simulink model "ADMIRE"  (R2021b)
settings: Solver=ode4  StartTime=0.0  StopTime=100  FixedStep=1e-2  RelTol=1e-3
undefined symbols (not defined in the file or in its folder): admireDB, Earth, WGS84
libraries: simulink_extras x112, simulink x27, aerolibutil x4, dspsigops x4, aerolibfltsims x3, sharedtransform x2, aerolibtransform2 x2, aerolibatmos2 x1, matrix_library x1, sharedutil x1, aerolibanimutils x1, vrlib x1
(part 15 of 15)

== system ADMIRE/Aircraft/Aerodynamics/YawMomentCoefficient/MachRegion3/Cymdr/Cymdr_ ==
  angleOfAttack_deg : Inport
  mach_nd : Inport  Port=2
  dR : Inport  Port=3
  qacorr : Inport  Port=4
  CYMDRAM_ALFA_M : Lookup_n-D  BreakpointsForDimension1=admireDB.aerodata_asym_ext.CYMDRAM.breakpoints.M  BreakpointsForDimension2=admireDB.aerodata_asym_ext.CYMDRAM.breakpoints.ALFA  BreakpointsForDimension3=[5, 7]  Table=admireDB.aerodata_asym_ext.CYMDRAM.newTable  ExtrapMethod=Clip  InternalRulePriority=Speed  RndMeth=Simplest  InputSameDT=on
      settings: InputPortMap=u0,u1
  CYMEDR_QA_M : Lookup_n-D  BreakpointsForDimension1=admireDB.aerodata_asym_ext.CYMEDR.breakpoints.M  BreakpointsForDimension2=admireDB.aerodata_asym_ext.CYMEDR.breakpoints.QA  BreakpointsForDimension3=[5, 7]  Table=admireDB.aerodata_asym_ext.CYMEDR.newTable  ExtrapMethod=Clip  InternalRulePriority=Speed  RndMeth=Simplest  InputSameDT=on
      settings: InputPortMap=u0,u1
  Degrees to Radians : simulink_extras/Transformations/Degrees to Radians
  Product : Product  Inputs=***
  Cymdr : Outport
  wires:
  Product/1 -> Cymdr/1
  CYMEDR_QA_M/1 -> Product/3
  qacorr/1 -> CYMEDR_QA_M/2
  mach_nd/1 -> CYMEDR_QA_M/1, CYMDRAM_ALFA_M/1
  Degrees to Radians/1 -> Product/2
  angleOfAttack_deg/1 -> CYMDRAM_ALFA_M/2
  CYMDRAM_ALFA_M/1 -> Product/1
  dR/1 -> Degrees to Radians/1

== system ADMIRE/Aircraft/Aerodynamics/YawMomentCoefficient/MachRegion3/Cymp/Cymp_ ==
  angleOfAttack_deg : Inport
  mach_nd : Inport  Port=2
  qacorr : Inport  Port=3
  pc : Inport  Port=4
  CYMEP_QA_M : Lookup_n-D  BreakpointsForDimension1=admireDB.aerodata_asym_ext.CYMEP.breakpoints.M  BreakpointsForDimension2=admireDB.aerodata_asym_ext.CYMEP.breakpoints.QA  BreakpointsForDimension3=[5, 7]  Table=admireDB.aerodata_asym_ext.CYMEP.newTable  ExtrapMethod=Clip  InternalRulePriority=Speed  RndMeth=Simplest  InputSameDT=on
      settings: InputPortMap=u0,u1
  CYMPAM_ALFA_M : Lookup_n-D  BreakpointsForDimension1=admireDB.aerodata_asym_ext.CYMPAM.breakpoints.M  BreakpointsForDimension2=admireDB.aerodata_asym_ext.CYMPAM.breakpoints.ALFA  BreakpointsForDimension3=[5, 7]  Table=admireDB.aerodata_asym_ext.CYMPAM.newTable  ExtrapMethod=Clip  InternalRulePriority=Speed  RndMeth=Simplest  InputSameDT=on
      settings: InputPortMap=u0,u1
  Product : Product
  Sum : Sum  Inputs=|++
  Cymp : Outport
  wires:
  qacorr/1 -> CYMEP_QA_M/2
  CYMEP_QA_M/1 -> Sum/2
  Sum/1 -> Product/1
  mach_nd/1 -> CYMPAM_ALFA_M/1, CYMEP_QA_M/1
  pc/1 -> Product/2
  Product/1 -> Cymp/1
  angleOfAttack_deg/1 -> CYMPAM_ALFA_M/2
  CYMPAM_ALFA_M/1 -> Sum/1

== system ADMIRE/Aircraft/Aerodynamics/YawMomentCoefficient/MachRegion3/Cymr/Cymr_ ==
  mach_nd : Inport
  angleOfAttack_deg : Inport  Port=2
  dN : Inport  Port=3
  qacorr : Inport  Port=4
  rc : Inport  Port=5
  CYMER_M_QA : Lookup_n-D  BreakpointsForDimension1=admireDB.aerodata_asym_ext.CYMER.breakpoints.QA  BreakpointsForDimension2=admireDB.aerodata_asym_ext.CYMER.breakpoints.M  BreakpointsForDimension3=[5, 7]  Table=admireDB.aerodata_asym_ext.CYMER.newTable  ExtrapMethod=Clip  InternalRulePriority=Speed  RndMeth=Simplest  InputSameDT=on
      settings: InputPortMap=u0,u1
  CYMRAM_M_ALFA_DN : Lookup_n-D  NumberOfTableDimensions=3  BreakpointsForDimension1=admireDB.aerodata_asym_ext.CYMRAM.breakpoints.M  BreakpointsForDimension2=admireDB.aerodata_asym_ext.CYMRAM.breakpoints.ALFA  BreakpointsForDimension3=admireDB.aerodata_asym_ext.CYMRAM.breakpoints.DN  Table=admireDB.aerodata_asym_ext.CYMRAM.newTable  ExtrapMethod=Clip  InternalRulePriority=Speed  RndMeth=Simplest  InputSameDT=on
      settings: InputPortMap=u0,u1,u2
  Product : Product  Inputs=***
  Cymr : Outport
  wires:
  CYMER_M_QA/1 -> Product/3
  qacorr/1 -> CYMER_M_QA/1
  dN/1 -> CYMRAM_M_ALFA_DN/3
  rc/1 -> Product/2
  Product/1 -> Cymr/1
  mach_nd/1 -> CYMRAM_M_ALFA_DN/1, CYMER_M_QA/2
  angleOfAttack_deg/1 -> CYMRAM_M_ALFA_DN/2
  CYMRAM_M_ALFA_DN/1 -> Product/1

== system ADMIRE/Aircraft/Aerodynamics/YawMomentCoefficient/MachRegion4/Cymbcai/Cymbcai_ ==
  CAI : Inport
  angleOfAttack_deg : Inport  Port=2
  angleOfSideslip_deg : Inport  Port=3
  CYMBCAI_CAI_ALFA : Lookup_n-D  BreakpointsForDimension1=admireDB.aerodata_asym_ext.CYMBCAI.breakpoints.ALFA  BreakpointsForDimension2=admireDB.aerodata_asym_ext.CYMBCAI.breakpoints.CAI  BreakpointsForDimension3=[5, 7]  Table=admireDB.aerodata_asym_ext.CYMBCAI.newTable  ExtrapMethod=Clip  InternalRulePriority=Speed  RndMeth=Simplest  InputSameDT=on
      settings: InputPortMap=u0,u1
  Degrees to Radians : simulink_extras/Transformations/Degrees to Radians
  Product : Product  Inputs=**
  Cymbcai : Outport
  wires:
  CAI/1 -> CYMBCAI_CAI_ALFA/2
  angleOfSideslip_deg/1 -> Degrees to Radians/1
  CYMBCAI_CAI_ALFA/1 -> Product/1
  angleOfAttack_deg/1 -> CYMBCAI_CAI_ALFA/1
  Degrees to Radians/1 -> Product/2
  Product/1 -> Cymbcai/1

== system ADMIRE/Aircraft/Aerodynamics/YawMomentCoefficient/MachRegion4/Cymbde/Cymbde_ ==
  angleOfAttack_deg : Inport
  dEI : Inport  Port=2
  angleOfSideslip_deg : Inport  Port=3
  dEY : Inport  Port=4
  eieff : Inport  Port=5
  eoeff : Inport  Port=6
  mach_nd : Inport  Port=7
  Abs : Abs
  CYMBKM_M : Lookup_n-D  NumberOfTableDimensions=1  BreakpointsForDimension1=admireDB.aerodata_asym_ext.CYMBKM.breakpoints.M  BreakpointsForDimension3=[5, 7]  Table=admireDB.aerodata_asym_ext.CYMBKM.newTable  ExtrapMethod=Clip  InternalRulePriority=Speed  RndMeth=Simplest  InputSameDT=on
  CYMDEB_ALFA_DE_BETA : Lookup_n-D  NumberOfTableDimensions=3  BreakpointsForDimension1=admireDB.aerodata_asym_ext.CYMDEB.breakpoints.ALFA  BreakpointsForDimension2=admireDB.aerodata_asym_ext.CYMDEB.breakpoints.DE  BreakpointsForDimension3=admireDB.aerodata_asym_ext.CYMDEB.breakpoints.BETA  Table=admireDB.aerodata_asym_ext.CYMDEB.newTable  ExtrapMethod=Clip  InternalRulePriority=Speed  RndMeth=Simplest  InputSameDT=on
      settings: InputPortMap=u0,u1,u2
  CYMDEB_ALFA_DE_BETA1 : Lookup_n-D  NumberOfTableDimensions=3  BreakpointsForDimension1=admireDB.aerodata_asym_ext.CYMDEB.breakpoints.ALFA  BreakpointsForDimension2=admireDB.aerodata_asym_ext.CYMDEB.breakpoints.DE  BreakpointsForDimension3=admireDB.aerodata_asym_ext.CYMDEB.breakpoints.BETA  Table=admireDB.aerodata_asym_ext.CYMDEB.newTable  ExtrapMethod=Clip  InternalRulePriority=Speed  RndMeth=Simplest  InputSameDT=on
      settings: InputPortMap=u0,u1,u2
  Product : Product  Inputs=**
  Product1 : Product  Inputs=**
  Product2 : Product  Inputs=***
  Sign : Signum
  Sum : Sum  Inputs=|++
  Cymbde : Outport
  wires:
  Product2/1 -> Cymbde/1
  dEI/1 -> CYMDEB_ALFA_DE_BETA/2
  angleOfSideslip_deg/1 -> Abs/1, Sign/1
  CYMDEB_ALFA_DE_BETA/1 -> Product/1
  eieff/1 -> Product/2
  dEY/1 -> CYMDEB_ALFA_DE_BETA1/2
  Abs/1 -> CYMDEB_ALFA_DE_BETA/3, CYMDEB_ALFA_DE_BETA1/3
  angleOfAttack_deg/1 -> CYMDEB_ALFA_DE_BETA/1, CYMDEB_ALFA_DE_BETA1/1
  CYMDEB_ALFA_DE_BETA1/1 -> Product1/1
  eoeff/1 -> Product1/2
  Product/1 -> Sum/1
  Product1/1 -> Sum/2
  Sum/1 -> Product2/1
  Sign/1 -> Product2/2
  CYMBKM_M/1 -> Product2/3
  mach_nd/1 -> CYMBKM_M/1

== system ADMIRE/Aircraft/Aerodynamics/YawMomentCoefficient/MachRegion4/Cymbdle/Cymbdle_ ==
  angleOfAttack_deg : Inport
  dEI : Inport  Port=2
  mach_nd : Inport  Port=3
  dEY : Inport  Port=4
  eieff : Inport  Port=5
  eoeff : Inport  Port=6
  angleOfSideslip_deg : Inport  Port=7
  dLE : Inport  Port=8
  CYMBDLE_ALFA_DE_M : Lookup_n-D  NumberOfTableDimensions=3  BreakpointsForDimension1=admireDB.aerodata_asym_ext.CYMBDLE.breakpoints.ALFA  BreakpointsForDimension2=admireDB.aerodata_asym_ext.CYMBDLE.breakpoints.DE  BreakpointsForDimension3=admireDB.aerodata_asym_ext.CYMBDLE.breakpoints.M  Table=admireDB.aerodata_asym_ext.CYMBDLE.newTable  ExtrapMethod=Clip  InternalRulePriority=Speed  RndMeth=Simplest  InputSameDT=on
      settings: InputPortMap=u0,u1,u2
  CYMBDLE_ALFA_DE_M1 : Lookup_n-D  NumberOfTableDimensions=3  BreakpointsForDimension1=admireDB.aerodata_asym_ext.CYMBDLE.breakpoints.ALFA  BreakpointsForDimension2=admireDB.aerodata_asym_ext.CYMBDLE.breakpoints.DE  BreakpointsForDimension3=admireDB.aerodata_asym_ext.CYMBDLE.breakpoints.M  Table=admireDB.aerodata_asym_ext.CYMBDLE.newTable  ExtrapMethod=Clip  InternalRulePriority=Speed  RndMeth=Simplest  InputSameDT=on
      settings: InputPortMap=u0,u1,u2
  Constant : Constant  Value=1/27
  Degrees to Radians : simulink_extras/Transformations/Degrees to Radians
  Product : Product  Inputs=**
  Product1 : Product  Inputs=**
  Product2 : Product  Inputs=****
  Sum : Sum  Inputs=|++
  Cymbdle : Outport
  wires:
  Product2/1 -> Cymbdle/1
  CYMBDLE_ALFA_DE_M/1 -> Product/1
  dEI/1 -> CYMBDLE_ALFA_DE_M/2
  eieff/1 -> Product/2
  mach_nd/1 -> CYMBDLE_ALFA_DE_M1/3, CYMBDLE_ALFA_DE_M/3
  angleOfAttack_deg/1 -> CYMBDLE_ALFA_DE_M1/1, CYMBDLE_ALFA_DE_M/1
  CYMBDLE_ALFA_DE_M1/1 -> Product1/1
  dEY/1 -> CYMBDLE_ALFA_DE_M1/2
  eoeff/1 -> Product1/2
  Product/1 -> Sum/1
  Product1/1 -> Sum/2
  Sum/1 -> Product2/2
  angleOfSideslip_deg/1 -> Degrees to Radians/1
  Degrees to Radians/1 -> Product2/1
  dLE/1 -> Product2/3
  Constant/1 -> Product2/4

== system ADMIRE/Aircraft/Aerodynamics/YawMomentCoefficient/MachRegion4/Cymbdn/Cymbdn_ ==
  angleOfAttack_deg : Inport
  dN : Inport  Port=2
  angleOfSideslip_deg : Inport  Port=3
  Abs : Abs
  CYMDNB_ALFA_DN_BETA : Lookup_n-D  NumberOfTableDimensions=3  BreakpointsForDimension1=admireDB.aerodata_asym_ext.CYMDNB.breakpoints.ALFA  BreakpointsForDimension2=admireDB.aerodata_asym_ext.CYMDNB.breakpoints.DN  BreakpointsForDimension3=admireDB.aerodata_asym_ext.CYMDNB.breakpoints.BETA  Table=admireDB.aerodata_asym_ext.CYMDNB.newTable  ExtrapMethod=Clip  InternalRulePriority=Speed  RndMeth=Simplest  InputSameDT=on
      settings: InputPortMap=u0,u1,u2
  Product : Product  Inputs=**
  Sign : Signum
  Cymbdn : Outport
  wires:
  Product/1 -> Cymbdn/1
  angleOfSideslip_deg/1 -> Sign/1, Abs/1
  angleOfAttack_deg/1 -> CYMDNB_ALFA_DN_BETA/1
  Sign/1 -> Product/2
  CYMDNB_ALFA_DN_BETA/1 -> Product/1
  dN/1 -> CYMDNB_ALFA_DN_BETA/2
  Abs/1 -> CYMDNB_ALFA_DN_BETA/3

== system ADMIRE/Aircraft/Aerodynamics/YawMomentCoefficient/MachRegion4/Cymbeta/Cymbeta_ ==
  angleOfSideslip_deg : Inport
  angleOfAttack_deg : Inport  Port=2
  mach_nd : Inport  Port=3
  qacorr : Inport  Port=4
  Abs : Abs
  CYMEB_QA_M : Lookup_n-D  BreakpointsForDimension1=admireDB.aerodata_asym_ext.CYMEB.breakpoints.M  BreakpointsForDimension2=admireDB.aerodata_asym_ext.CYMEB.breakpoints.QA  BreakpointsForDimension3=[5, 7]  Table=admireDB.aerodata_asym_ext.CYMEB.newTable  ExtrapMethod=Clip  InternalRulePriority=Speed  RndMeth=Simplest  InputSameDT=on
      settings: InputPortMap=u0,u1
  CYMMAB_BETA_ALFA_M : Lookup_n-D  NumberOfTableDimensions=3  BreakpointsForDimension1=admireDB.aerodata_asym_ext.CYMMAB.breakpoints.BETA  BreakpointsForDimension2=admireDB.aerodata_asym_ext.CYMMAB.breakpoints.ALFA  BreakpointsForDimension3=admireDB.aerodata_asym_ext.CYMMAB.breakpoints.M  Table=admireDB.aerodata_asym_ext.CYMMAB.newTable  ExtrapMethod=Clip  InternalRulePriority=Speed  RndMeth=Simplest  InputSameDT=on
      settings: InputPortMap=u0,u1,u2
  Degrees to Radians : simulink_extras/Transformations/Degrees to Radians
  Product : Product  Inputs=**
  Product1 : Product  Inputs=**
  Sign : Signum
  Sum : Sum  Inputs=|++
  Cymbeta : Outport
  wires:
  CYMMAB_BETA_ALFA_M/1 -> Product/2
  angleOfAttack_deg/1 -> CYMMAB_BETA_ALFA_M/2
  Sign/1 -> Product/1
  Product/1 -> Sum/1
  Sum/1 -> Cymbeta/1
  angleOfSideslip_deg/1 -> Sign/1, Degrees to Radians/1, Abs/1
  mach_nd/1 -> CYMMAB_BETA_ALFA_M/3, CYMEB_QA_M/1
  CYMEB_QA_M/1 -> Product1/1
  qacorr/1 -> CYMEB_QA_M/2
  Degrees to Radians/1 -> Product1/2
  Abs/1 -> CYMMAB_BETA_ALFA_M/1
  Product1/1 -> Sum/2

== system ADMIRE/Aircraft/Aerodynamics/YawMomentCoefficient/MachRegion4/Cymbetad/Cymbetad_ ==
  angleOfAttack_deg : Inport
  mach_nd : Inport  Port=2
  betad : Inport  Port=3
  CYMBDH_ALFA_M : Lookup_n-D  BreakpointsForDimension1=admireDB.aerodata_asym_ext.CYMBDH.breakpoints.M  BreakpointsForDimension2=admireDB.aerodata_asym_ext.CYMBDH.breakpoints.ALFA  BreakpointsForDimension3=[5, 7]  Table=admireDB.aerodata_asym_ext.CYMBDH.newTable  ExtrapMethod=Clip  InternalRulePriority=Speed  RndMeth=Simplest  InputSameDT=on
      settings: InputPortMap=u0,u1
  Product : Product  Inputs=**
  Cymbetad : Outport
  wires:
  mach_nd/1 -> CYMBDH_ALFA_M/1
  angleOfAttack_deg/1 -> CYMBDH_ALFA_M/2
  CYMBDH_ALFA_M/1 -> Product/1
  Product/1 -> Cymbetad/1
  betad/1 -> Product/2

== system ADMIRE/Aircraft/Aerodynamics/YawMomentCoefficient/MachRegion4/Cymblg/Cymblg_ ==
  angleOfSideslip_deg : Inport
  dLG : Inport  Port=2
  angleOfAttack_deg : Inport  Port=3
  CYMBLST_NG_DOOR_ALFA : Lookup_n-D  BreakpointsForDimension1=admireDB.aerodata_asym_ext.CYMBLST.breakpoints.ALFA  BreakpointsForDimension2=admireDB.aerodata_asym_ext.CYMBLST.breakpoints.NG_DOOR  BreakpointsForDimension3=[5, 7]  Table=admireDB.aerodata_asym_ext.CYMBLST.newTable  ExtrapMethod=Clip  InternalRulePriority=Speed  RndMeth=Simplest  InputSameDT=on
      settings: InputPortMap=u0,u1
  Degrees to Radians : simulink_extras/Transformations/Degrees to Radians
  Product : Product  Inputs=3
  Cymblg : Outport
  wires:
  CYMBLST_NG_DOOR_ALFA/1 -> Product/3
  Product/1 -> Cymblg/1
  dLG/1 -> CYMBLST_NG_DOOR_ALFA/2, Product/2
  angleOfSideslip_deg/1 -> Degrees to Radians/1
  angleOfAttack_deg/1 -> CYMBLST_NG_DOOR_ALFA/1
  Degrees to Radians/1 -> Product/1

== system ADMIRE/Aircraft/Aerodynamics/YawMomentCoefficient/MachRegion4/Cymdai/Cymdai_ ==
  dAI : Inport
  angleOfAttack_deg : Inport  Port=2
  dEI : Inport  Port=3
  mach_nd : Inport  Port=4
  eieff : Inport  Port=5
  qacorr : Inport  Port=6
  CYMDA_ALFA_DE_M : Lookup_n-D  NumberOfTableDimensions=3  BreakpointsForDimension1=admireDB.aerodata_asym_ext.CYMDA.breakpoints.ALFA  BreakpointsForDimension2=admireDB.aerodata_asym_ext.CYMDA.breakpoints.DE  BreakpointsForDimension3=admireDB.aerodata_asym_ext.CYMDA.breakpoints.M  Table=admireDB.aerodata_asym_ext.CYMDA.newTable  ExtrapMethod=Clip  InternalRulePriority=Speed  RndMeth=Simplest  InputSameDT=on
      settings: InputPortMap=u0,u1,u2
  CYMEDAI_QA_M : Lookup_n-D  BreakpointsForDimension1=admireDB.aerodata_asym_ext.CYMEDAI.breakpoints.M  BreakpointsForDimension2=admireDB.aerodata_asym_ext.CYMEDAI.breakpoints.QA  BreakpointsForDimension3=[5, 7]  Table=admireDB.aerodata_asym_ext.CYMEDAI.newTable  ExtrapMethod=Clip  InternalRulePriority=Speed  RndMeth=Simplest  InputSameDT=on
      settings: InputPortMap=u0,u1
  Degrees to Radians : simulink_extras/Transformations/Degrees to Radians
  Product1 : Product  Inputs=3
  Product2 : Product  Inputs=**
  Cymdai : Outport
  wires:
  qacorr/1 -> CYMEDAI_QA_M/2
  eieff/1 -> Product1/2
  Product2/1 -> Cymdai/1
  dAI/1 -> Degrees to Radians/1
  dEI/1 -> CYMDA_ALFA_DE_M/2
  mach_nd/1 -> CYMDA_ALFA_DE_M/3, CYMEDAI_QA_M/1
  angleOfAttack_deg/1 -> CYMDA_ALFA_DE_M/1
  CYMDA_ALFA_DE_M/1 -> Product1/3
  Degrees to Radians/1 -> Product1/1
  CYMEDAI_QA_M/1 -> Product2/2
  Product1/1 -> Product2/1

== system ADMIRE/Aircraft/Aerodynamics/YawMomentCoefficient/MachRegion4/Cymday/Cymday_ ==
  angleOfAttack_deg : Inport
  dEY : Inport  Port=2
  mach_nd : Inport  Port=3
  qacorr : Inport  Port=4
  eoeff : Inport  Port=5
  dAY : Inport  Port=6
  CYMDA_ALFA_DE_M : Lookup_n-D  NumberOfTableDimensions=3  BreakpointsForDimension1=admireDB.aerodata_asym_ext.CYMDA.breakpoints.ALFA  BreakpointsForDimension2=admireDB.aerodata_asym_ext.CYMDA.breakpoints.DE  BreakpointsForDimension3=admireDB.aerodata_asym_ext.CYMDA.breakpoints.M  Table=admireDB.aerodata_asym_ext.CYMDA.newTable  ExtrapMethod=Clip  InternalRulePriority=Speed  RndMeth=Simplest  InputSameDT=on
      settings: InputPortMap=u0,u1,u2
  CYMEDAY_QA_M : Lookup_n-D  BreakpointsForDimension1=admireDB.aerodata_asym_ext.CYMEDAY.breakpoints.M  BreakpointsForDimension2=admireDB.aerodata_asym_ext.CYMEDAY.breakpoints.QA  BreakpointsForDimension3=[5, 7]  Table=admireDB.aerodata_asym_ext.CYMEDAY.newTable  ExtrapMethod=Clip  InternalRulePriority=Speed  RndMeth=Simplest  InputSameDT=on
      settings: InputPortMap=u0,u1
  Degrees to Radians : simulink_extras/Transformations/Degrees to Radians
  Product : Product  Inputs=**
  Product1 : Product
  Sum : Sum  Inputs=|++
  Cymday : Outport
  wires:
  qacorr/1 -> CYMEDAY_QA_M/2
  Product1/1 -> Cymday/1
  Sum/1 -> Product1/1
  Degrees to Radians/1 -> Product1/2
  dAY/1 -> Degrees to Radians/1
  Product/1 -> Sum/1
  CYMEDAY_QA_M/1 -> Sum/2
  mach_nd/1 -> CYMDA_ALFA_DE_M/3, CYMEDAY_QA_M/1
  eoeff/1 -> Product/2
  CYMDA_ALFA_DE_M/1 -> Product/1
  angleOfAttack_deg/1 -> CYMDA_ALFA_DE_M/1
  dEY/1 -> CYMDA_ALFA_DE_M/2

== system ADMIRE/Aircraft/Aerodynamics/YawMomentCoefficient/MachRegion4/Cymdna/Cymdna_ ==
  angleOfAttack_deg : Inport
  mach_nd : Inport  Port=2
  dNA : Inport  Port=3
  CYMDNAAM_ALFA_M : Lookup_n-D  BreakpointsForDimension1=admireDB.aerodata_asym_ext.CYMDNAAM.breakpoints.M  BreakpointsForDimension2=admireDB.aerodata_asym_ext.CYMDNAAM.breakpoints.ALFA  BreakpointsForDimension3=[5, 7]  Table=admireDB.aerodata_asym_ext.CYMDNAAM.newTable  ExtrapMethod=Clip  InternalRulePriority=Speed  RndMeth=Simplest  InputSameDT=on
      settings: InputPortMap=u0,u1
  Degrees to Radians : simulink_extras/Transformations/Degrees to Radians
  Product : Product  Inputs=**
  Cymdna : Outport
  wires:
  mach_nd/1 -> CYMDNAAM_ALFA_M/1
  angleOfAttack_deg/1 -> CYMDNAAM_ALFA_M/2
  CYMDNAAM_ALFA_M/1 -> Product/1
  Degrees to Radians/1 -> Product/2
  dNA/1 -> Degrees to Radians/1
  Product/1 -> Cymdna/1

== system ADMIRE/Aircraft/Aerodynamics/YawMomentCoefficient/MachRegion4/Cymdr/Cymdr_ ==
  angleOfAttack_deg : Inport
  mach_nd : Inport  Port=2
  dR : Inport  Port=3
  qacorr : Inport  Port=4
  CYMDRAM_ALFA_M : Lookup_n-D  BreakpointsForDimension1=admireDB.aerodata_asym_ext.CYMDRAM.breakpoints.M  BreakpointsForDimension2=admireDB.aerodata_asym_ext.CYMDRAM.breakpoints.ALFA  BreakpointsForDimension3=[5, 7]  Table=admireDB.aerodata_asym_ext.CYMDRAM.newTable  ExtrapMethod=Clip  InternalRulePriority=Speed  RndMeth=Simplest  InputSameDT=on
      settings: InputPortMap=u0,u1
  CYMEDR_QA_M : Lookup_n-D  BreakpointsForDimension1=admireDB.aerodata_asym_ext.CYMEDR.breakpoints.M  BreakpointsForDimension2=admireDB.aerodata_asym_ext.CYMEDR.breakpoints.QA  BreakpointsForDimension3=[5, 7]  Table=admireDB.aerodata_asym_ext.CYMEDR.newTable  ExtrapMethod=Clip  InternalRulePriority=Speed  RndMeth=Simplest  InputSameDT=on
      settings: InputPortMap=u0,u1
  Degrees to Radians : simulink_extras/Transformations/Degrees to Radians
  Product : Product  Inputs=***
  Cymdr : Outport
  wires:
  dR/1 -> Degrees to Radians/1
  CYMDRAM_ALFA_M/1 -> Product/1
  angleOfAttack_deg/1 -> CYMDRAM_ALFA_M/2
  Degrees to Radians/1 -> Product/2
  mach_nd/1 -> CYMEDR_QA_M/1, CYMDRAM_ALFA_M/1
  qacorr/1 -> CYMEDR_QA_M/2
  CYMEDR_QA_M/1 -> Product/3
  Product/1 -> Cymdr/1

== system ADMIRE/Aircraft/Aerodynamics/YawMomentCoefficient/MachRegion4/Cymp/Cymp_ ==
  angleOfAttack_deg : Inport
  mach_nd : Inport  Port=2
  qacorr : Inport  Port=3
  pc : Inport  Port=4
  CYMEP_QA_M : Lookup_n-D  BreakpointsForDimension1=admireDB.aerodata_asym_ext.CYMEP.breakpoints.M  BreakpointsForDimension2=admireDB.aerodata_asym_ext.CYMEP.breakpoints.QA  BreakpointsForDimension3=[5, 7]  Table=admireDB.aerodata_asym_ext.CYMEP.newTable  ExtrapMethod=Clip  InternalRulePriority=Speed  RndMeth=Simplest  InputSameDT=on
      settings: InputPortMap=u0,u1
  CYMPAM_ALFA_M : Lookup_n-D  BreakpointsForDimension1=admireDB.aerodata_asym_ext.CYMPAM.breakpoints.M  BreakpointsForDimension2=admireDB.aerodata_asym_ext.CYMPAM.breakpoints.ALFA  BreakpointsForDimension3=[5, 7]  Table=admireDB.aerodata_asym_ext.CYMPAM.newTable  ExtrapMethod=Clip  InternalRulePriority=Speed  RndMeth=Simplest  InputSameDT=on
      settings: InputPortMap=u0,u1
  Product : Product
  Sum : Sum  Inputs=|++
  Cymp : Outport
  wires:
  qacorr/1 -> CYMEP_QA_M/2
  CYMEP_QA_M/1 -> Sum/2
  Sum/1 -> Product/1
  CYMPAM_ALFA_M/1 -> Sum/1
  angleOfAttack_deg/1 -> CYMPAM_ALFA_M/2
  Product/1 -> Cymp/1
  pc/1 -> Product/2
  mach_nd/1 -> CYMPAM_ALFA_M/1, CYMEP_QA_M/1

== system ADMIRE/Aircraft/Aerodynamics/YawMomentCoefficient/MachRegion4/Cymr/Cymr_ ==
  mach_nd : Inport
  angleOfAttack_deg : Inport  Port=2
  dN : Inport  Port=3
  qacorr : Inport  Port=4
  rc : Inport  Port=5
  CYMER_M_QA : Lookup_n-D  BreakpointsForDimension1=admireDB.aerodata_asym_ext.CYMER.breakpoints.QA  BreakpointsForDimension2=admireDB.aerodata_asym_ext.CYMER.breakpoints.M  BreakpointsForDimension3=[5, 7]  Table=admireDB.aerodata_asym_ext.CYMER.newTable  ExtrapMethod=Clip  InternalRulePriority=Speed  RndMeth=Simplest  InputSameDT=on
      settings: InputPortMap=u0,u1
  CYMRAM_M_ALFA_DN : Lookup_n-D  NumberOfTableDimensions=3  BreakpointsForDimension1=admireDB.aerodata_asym_ext.CYMRAM.breakpoints.M  BreakpointsForDimension2=admireDB.aerodata_asym_ext.CYMRAM.breakpoints.ALFA  BreakpointsForDimension3=admireDB.aerodata_asym_ext.CYMRAM.breakpoints.DN  Table=admireDB.aerodata_asym_ext.CYMRAM.newTable  ExtrapMethod=Clip  InternalRulePriority=Speed  RndMeth=Simplest  InputSameDT=on
      settings: InputPortMap=u0,u1,u2
  Product : Product  Inputs=***
  Cymr : Outport
  wires:
  qacorr/1 -> CYMER_M_QA/1
  CYMRAM_M_ALFA_DN/1 -> Product/1
  angleOfAttack_deg/1 -> CYMRAM_M_ALFA_DN/2
  mach_nd/1 -> CYMER_M_QA/2, CYMRAM_M_ALFA_DN/1
  Product/1 -> Cymr/1
  rc/1 -> Product/2
  dN/1 -> CYMRAM_M_ALFA_DN/3
  CYMER_M_QA/1 -> Product/3
